simulink model "Simulink_Model-bugged"  (R2021a)
settings: Solver=VariableStepAuto  StartTime=0.0  StopTime=inf  FixedStep=1  RelTol=1e-3
model workspace (MAT data in the model file):
  M = 1200
  R = 1
libraries: simulink x2, pid_lib x1
settings Model: EnablePacing=on  Creator=matteopenlington  LastModifiedBy=matteopenlington
settings DebuggingCC: UnderSpecifiedDimensionMsg=warning

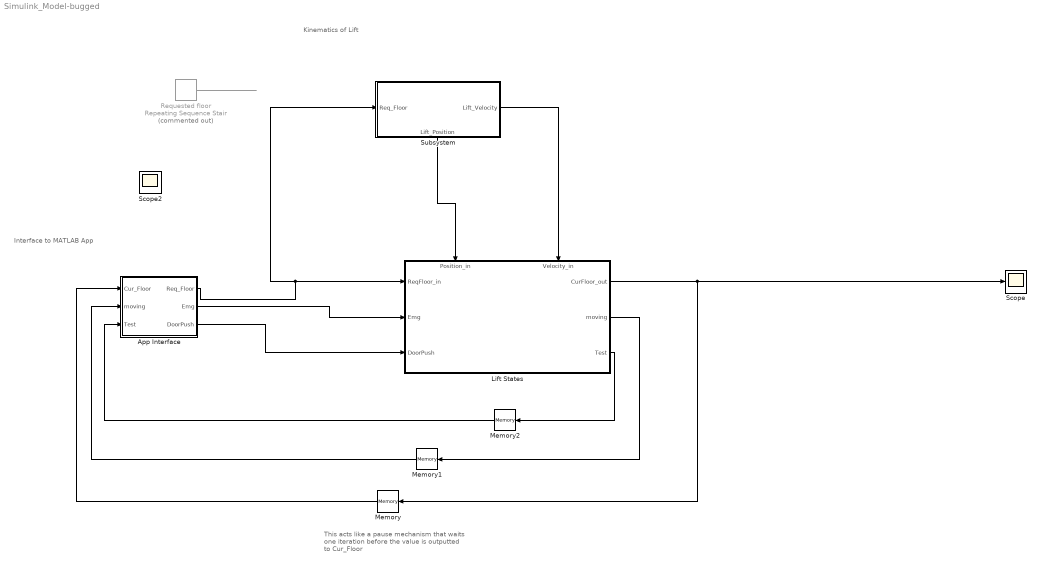
== system Simulink_Model-bugged ==
  note: This acts like a pause mechanism that waits one iteration before the value is outputted to Cur_Floor
  note: Interface to MATLAB App
  note: Kinematics of Lift
  App Interface : Stateflow chart  TreatAsAtomicUnit=on
  Lift States : Stateflow chart  TreatAsAtomicUnit=on
      settings: PortSchema="{\"entries\":[{\"content\":{\"sides\":[{\"content\":{\"connectorIds\":[\"In1\",\"In2\",\"In3\"]},\"type\":\"ConnectorPlacement.EquallySpacedRectSide\",\"uuid\":\"bd67e075-ced7-4894-beb9-3d24b34d513a\"},{\"content\":{\"connectorIds\":[\"Out1\",\"Out2\",\"Out3\"],\"side\":\"RIGHT\"},\"type\":\"ConnectorPlacement.EquallySpacedRectSide\",\"uuid\":\"62974800-2f1d-440c-84a5-b13d0b321f49\"},{\"content\":{\"connectorIds\":[\"In4\",\"In5\"],\"side\":\"TOP\"},\"type\":\"ConnectorPlacement.EquallySpacedRectSide\",\"uuid\":\"b0ebe389-7aaa-432d-aca6-247e3589a149\"}]},\"type\":\"ConnectorPlacement.EquallySpacedConnector\",\"uuid\":\"bed4184c-0ba6-4939-b370-ce80092994a7\"}],\"packageUris\":[\"http://schema.mathworks.com/mf0/Connector/R2020b\"],\"version\":\"1.0\"}"
  Memory : Memory
  Memory1 : Memory
  Memory2 : Memory
  Requested floor : simulink/Sources/Repeating Sequence Stair  Commented=on  OutValues=[2:8 5 2 8 7 1].'  tsamp=30  OutMin=[]  OutMax=[]  OutDataTypeStr=double  OutputDataTypeScalingMode=double  OutDataType=fixdt(0,8)  ConRadixGroup=Best Precision: Vector-wise  OutScaling=2^-12
  Scope : Scope
  Subsystem : Subsystem
      settings: PortSchema="{\"entries\":[{\"content\":{\"sides\":[{\"content\":{\"connectorIds\":[\"In1\"]},\"type\":\"ConnectorPlacement.EquallySpacedRectSide\",\"uuid\":\"5720384a-5b6b-4c8f-827c-e4dc33621555\"},{\"content\":{\"connectorIds\":[\"Out1\"],\"side\":\"RIGHT\"},\"type\":\"ConnectorPlacement.EquallySpacedRectSide\",\"uuid\":\"bb3a0671-b228-450f-9a0a-fbe23ffb3ccb\"},{\"content\":{\"connectorIds\":[],\"side\":\"TOP\"},\"type\":\"ConnectorPlacement.EquallySpacedRectSide\",\"uuid\":\"52cff964-e53a-4485-8402-576deae0ccd6\"},{\"content\":{\"connectorIds\":[\"Out2\"],\"side\":\"BOTTOM\"},\"type\":\"ConnectorPlacement.EquallySpacedRectSide\",\"uuid\":\"59af7eeb-6d0a-46f8-956e-aa24ce8e32b3\"}]},\"type\":\"ConnectorPlacement.EquallySpacedConnector\",\"uuid\":\"27d75544-d276-4748-ba1d-01bc4bb5bd0a\"}],\"packageUris\":[\"http://schema.mathworks.com/mf0/Connector/R2020b\"],\"version\":\"1.0\"}"
  Scope2 : Scope
  wires:
  Memory/1 -> App Interface/1(Cur_Floor)
  Lift States/1(CurFloor_out) -> Memory/1, Scope/1
  App Interface/2(Emg) -> Lift States/2(Emg)
  Lift States/2(moving) -> Memory1/1
  Memory1/1 -> App Interface/2(moving)
  App Interface/3(DoorPush) -> Lift States/3(DoorPush)
  Lift States/3(Test) -> Memory2/1
  Memory2/1 -> App Interface/3(Test)
  Requested floor/1 -> ?
  App Interface/1(Req_Floor) -> Lift States/1(ReqFloor_in), Subsystem/1(Req_Floor)
  Subsystem/2(Lift_Position) -> Lift States/4(Position_in)
  Subsystem/1(Lift_Velocity) -> Lift States/5(Velocity_in)

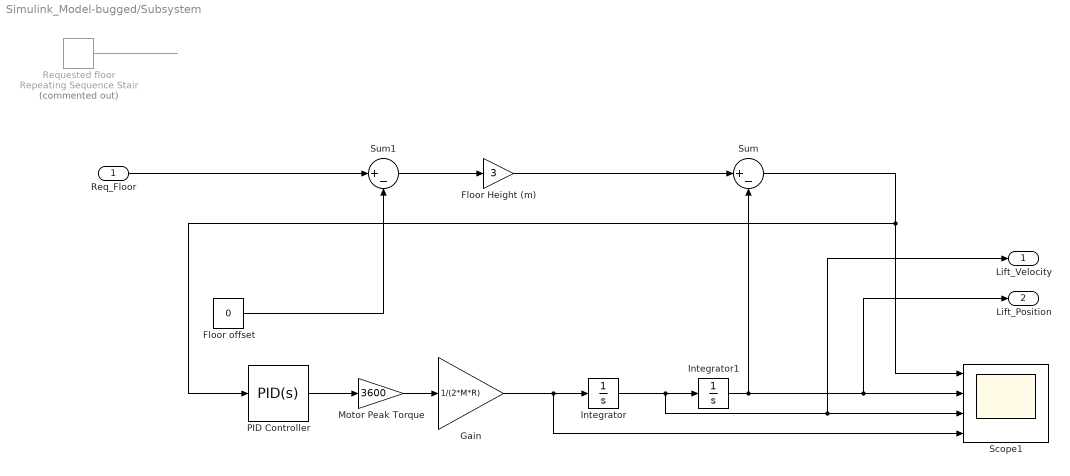
== system Simulink_Model-bugged/Subsystem ==
  Req_Floor : Inport
  Floor Height (m) : Gain  Gain=3
  Floor offset : Constant  Value=0
  Gain : Gain  Gain=1/(2*M*R)
  Integrator : Integrator
  Integrator1 : Integrator
  Motor Peak Torque : Gain  Gain=3600
  PID Controller : pid_lib/PID Controller  Controller=PID  Form=Parallel  TimeDomain=Continuous-time  UseExternalTs=off  SampleTime=-1  IntegratorMethod=Forward Euler  FilterMethod=Forward Euler  ControllerParametersSource=internal  P=1  I=0  D=2  UseFilter=on  N=5.45  TunerSelectOption=Transfer Function Based (PID Tuner App)  InitialConditionSource=internal  InitialConditionForIntegrator=0  InitialConditionForFilter=0  DifferentiatorICPrevScaledInput=0  ExternalReset=none  TrackingMode=off  Kt=1  LimitOutput=on  SatLimitsSource=internal  UpperSaturationLimit=1  LowerSaturationLimit=-1  LinearizeAsGain=on  AntiWindupMode=none  Kb=1  POutMin=[]  POutMax=[]  IOutMin=[]  IOutMax=[]  DOutMin=[]  DOutMax=[]  NOutMin=[]  NOutMax=[]  SumOutMin=[]  SumOutMax=[]  SaturationOutMin=[]  SaturationOutMax=[]  PParamMin=[]  PParamMax=[]  IParamMin=[]  IParamMax=[]  DParamMin=[]  DParamMax=[]  NParamMin=[]  NParamMax=[]  KbParamMin=[]  KbParamMax=[]  KtParamMin=[]  KtParamMax=[]  KbOutMin=[]  KbOutMax=[]  KtOutMin=[]  KtOutMax=[]  IntegratorOutMin=[]  IntegratorOutMax=[]  FilterOutMin=[]  FilterOutMax=[]  SumI1OutMin=[]  SumI1OutMax=[]  SumI2OutMin=[]  SumI2OutMax=[]  SumI3OutMin=[]  SumI3OutMax=[]  SumI4OutMin=[]  SumI4OutMax=[]  SumDOutMin=[]  SumDOutMax=[]  DifferentiatorOutMin=[]  DifferentiatorOutMax=[]  FilterDiffOutCoefMin=[]  FilterDiffOutCoefMax=[]  ReciprocalOutMin=[]  ReciprocalOutMax=[]  SumDenOutMin=[]  SumDenOutMax=[]  SumNumOutMin=[]  SumNumOutMax=[]  DivideOutMin=[]  DivideOutMax=[]  UdiffTsProdOutMin=[]  UdiffTsProdOutMax=[]  NTsProdOutMin=[]  NTsProdOutMax=[]  UintegralTsProdOutMin=[]  UintegralTsProdOutMax=[]  UngainTsProdOutMin=[]  UngainTsProdOutMax=[]  IntegratorContinuousStateAttributes=''  IntegratorStateMustResolveToSignalObject=off  IntegratorRTWStateStorageClass=Auto  FilterContinuousStateAttributes=''  FilterStateMustResolveToSignalObject=off  FilterRTWStateStorageClass=Auto  ParallelPVariant=InternalParameters  IdealPVariant=Disabled  IVariant=InternalParameters  DVariant=InternalParameters  IntegratorVariant=Continuous  SatVariant=Enabled  AWVariant=Passthrough  PCopyVariant=Disabled  TRVariant=Disabled  FdbkBlocksVariant=Forward  IdealPFdbkVariant=Disabled  SatFdbkVariant=Disabled  DerivativeFilterVariant=ContFilter  NVariant=InternalParameters  NCopyVariant=Disabled  FilterICVariant=InternalICsFilter  IntegratorICVariant=InternalICs  ExternalResetVariant=Disabled  TRSumVariant=Passthrough  SumFdbkVariant=Disabled  SumVariant=Sum_PID  TsampFilterVariant=InternalTs  TsampNgainVariant=Passthrough  TsampIntegralVariant=Passthrough  ExternalSaturationOutDataTypeStr=Inherit: Same as second input
  Requested floor : simulink/Sources/Repeating Sequence Stair  Commented=on  OutValues=[2:8 5 2 8 7 1].'  tsamp=30  OutMin=[]  OutMax=[]  OutDataTypeStr=double  OutputDataTypeScalingMode=double  OutDataType=fixdt(0,8)  ConRadixGroup=Best Precision: Vector-wise  OutScaling=2^-12
  Scope1 : Scope  NumInputPorts=4
  Sum : Sum  Inputs=|+-
  Sum1 : Sum  Inputs=|+-
  Lift_Velocity : Outport
  Lift_Position : Outport  Port=2
  wires:
  Requested floor/1 -> ?
  Req_Floor/1 -> Sum1/1
  Gain/1 -> Scope1/4, Integrator/1
  Sum/1 -> PID Controller/1, Scope1/1
  PID Controller/1 -> Motor Peak Torque/1
  Floor Height (m)/1 -> Sum/1
  Sum1/1 -> Floor Height (m)/1
  Integrator/1 -> Integrator1/1, Lift_Velocity/1, Scope1/3
  Integrator1/1 -> Sum/2, Lift_Position/1, Scope1/2
  Motor Peak Torque/1 -> Gain/1
  Floor offset/1 -> Sum1/2

== stateflow chart Simulink_Model-bugged/App Interface ==
  state InterfaceFromApp
    en:
    coder.extrinsic('AppWSimulink', 'updateCounter', 'Logic', 'Emergency', 'DoorOperation', 'updateDoorStatus');
    app = AppWSimulink(this);
    %Req_Floor = 2;
    initialiseData();
    Logic(app,Req_Floor);
    Emergency(app,Emg);
    DoorOperation(app, DoorPush)
    du:
    if hasChanged(Cur_Floor)
    updateCounter(app, Cur_Floor, Test, Req_Floor);
    end
    if isequal(Cur_Floor, Req_Floor)
    updateDoorStatus(app,Test);
    end
    if (Emg == 1)
    Reset;
    end
    state initialiseData [function]
      (default) -> (junction 12) : {
          | %CurFloor = 0;
          | Req_Floor = 0;
          | Emg = 0;
          | DoorPush =0;
          | }
    state Reset [function]
      (default) -> (junction 119) : {
          | Req_Floor = -10;
          | DoorPush =3;
          | }
  (default) -> InterfaceFromApp
  data: app local; Cur_Floor input; Req_Floor output; Emg output; moving input; DoorPush output; Test input

== stateflow chart Simulink_Model-bugged/Lift States ==
  state No_Error2
    entry:
    CurFloor = 0;
    door = 0;
    hasOpened = 1;
    doorClose = 0;
    state Motion [group]
      state MovingUp
        entry:
        moving = 1;
        CurFloor = CurFloor +1;
        exit:
        moving = 0;
      state MovingDown
        entry:
        moving = 1;
        exit:
        CurFloor = CurFloor - 1;
        moving =0;
    state Not_Moving
      entry:
      CurFloor_out = CurFloor;
      NxtFloor;
      Test = DoorPush;
      state NxtFloor [function]
        (default) -> (junction 212)
        (junction 212) -> (junction 213) [order 1] : [isempty(ReqFloor_in)]{ReqFloor = -10}
        (junction 212) -> (junction 214) [order 2] : {ReqFloor = ReqFloor_in;}
        (junction 213) -> (junction 215)
        (junction 214) -> (junction 215)
      state Idle
        en:
      state Doors
        state DoorClosed
          entry:
          Test =3;
          pause(2);
          doorClose = 1;
        state DoorOpening
          en:
          door = 0;
          doorClose = 0;
          Test = 0
          du:
          OpOpening;
        state DoorClosing
          en:
          ObjectDetection;
          Test = 2;
          du:
          ObjectDetection;
          OpClosing;
        state DoorOpen
          entry:
          Test = 1;
          hasOpened = 1;
        DoorOpening -> DoorOpen : [door >= 1]
        DoorClosing -> DoorClosed : [door <= 0]
        DoorOpen -> DoorClosing : after(2,sec)
      (default) -> Idle
      Idle -> DoorOpening [order 1] : [ReqFloor == CurFloor && hasOpened == 0]
    state OpOpening [function]
      (default) -> (junction 231) : [door <= 1]{door = door + 0.1;}
    state ObjectDetection [function]
      (default) -> (junction 234)
      (junction 234) -> (junction 235) [order 1] : [isempty(ReqFloor_in)]{ReqFloor = -10}
      (junction 234) -> (junction 236) [order 2] : {ReqFloor = ReqFloor_in;}
      (junction 235) -> (junction 237)
      (junction 236) -> (junction 237)
    state OpClosing [function]
      (default) -> (junction 244) : {door = door - 0.1;}
    (default) -> Not_Moving
    Not_Moving -> MovingUp [order 1] : [ReqFloor > CurFloor && door == 0]{hasOpened = 0}
    MovingUp -> Not_Moving : after(2,sec)
    Idle -> (junction 192) [order 2]
    (junction 192) -> (junction 193)
    MovingDown -> Not_Moving : after(2,sec)
    (junction 193) -> Not_Moving : after(0.001,sec)
    (junction 194) -> (junction 193)
    Not_Moving -> MovingDown [order 2] : [-2 < ReqFloor && ReqFloor < CurFloor && door == 0]{hasOpened = 0}
    Doors -> (junction 194) : [doorClose == 1]
  state Emergency
    en:
    Test = 0;
    hasOpened = 0;
  (default) -> No_Error2
  No_Error2 -> Emergency : [Emg == 1]
  Emergency -> No_Error2 : [Emg  == 0]
  data: Door local; Sensor local =0; CurFloor local; ReqFloor_in input; CurFloor_out output; ReqFloor local; Emg input; moving output; DoorPush input; door local; Test output; hasOpened local; doorClose local; Position_in input; Position local; Velocity local; Velocity_in input
